simulink model "im_model_1"  (R2022b)
settings: Solver=VariableStepAuto  StartTime=0.0  StopTime=0.5  RelTol=1e-3
values from neighbouring files (symbols this model uses):
  B = 0.00825    [IM_System_1.m]    (also in IM_System_2.m; IM_System_3.m; IM_System_noPU_4p2p2kw.m; IM_System_noPU_4p2p2kw_1.m)
  D = Ls*Lr - Lm^2    (= 0.000595276666667)    [IM_System_1.m]    (also in IM_System_2.m; IM_System_3.m; IM_System_noPU_4p2p2kw.m; IM_System_noPU_4p2p2kw_1.m)
  J = 0.013    [IM_System_1.m]    (also in IM_System_2.m; IM_System_3.m; IM_System_noPU_4p2p2kw.m; IM_System_noPU_4p2p2kw_1.m)
  Lm = 0.245/3    (= 0.0816666666667)    [IM_System_1.m]    (also in IM_System_2.m; IM_System_3.m; IM_System_noPU_4p2p2kw.m; IM_System_noPU_4p2p2kw_1.m)
  Lr = Ls    (= 0.0852333333333)    [IM_System_1.m]    (also in IM_System_2.m; IM_System_3.m; IM_System_noPU_4p2p2kw.m; IM_System_noPU_4p2p2kw_1.m)
  Ls = 0.2557/3    (= 0.0852333333333)    [IM_System_1.m]    (also in IM_System_2.m; IM_System_3.m; IM_System_noPU_4p2p2kw.m; IM_System_noPU_4p2p2kw_1.m)
  pole = 4    [im_params.m]
  Rr = 1.83/3    (= 0.61)    [IM_System_1.m]    (also in IM_System_2.m; IM_System_3.m; IM_System_noPU_4p2p2kw.m; IM_System_noPU_4p2p2kw_1.m)
  Rs = 2.5/3    (= 0.833333333333)    [IM_System_1.m]    (also in IM_System_2.m; IM_System_3.m; IM_System_noPU_4p2p2kw.m; IM_System_noPU_4p2p2kw_1.m)
  w = w + iq_err*dt    (= -0.00016)    [IM_System_1.m]    (also in IM_System_2.m = -2e-05; IM_System_3.m = -2.2624e-05; IM_System_noPU_4p2p2kw.m = 0; IM_System_noPU_4p2p2kw_1.m = 0)
settings Model: Creator=jack  LastModifiedBy=jack

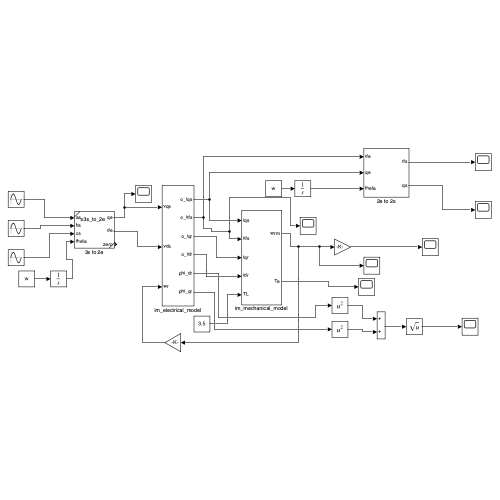
[thumbnail: Simulink's stored preview of the top-level diagram]
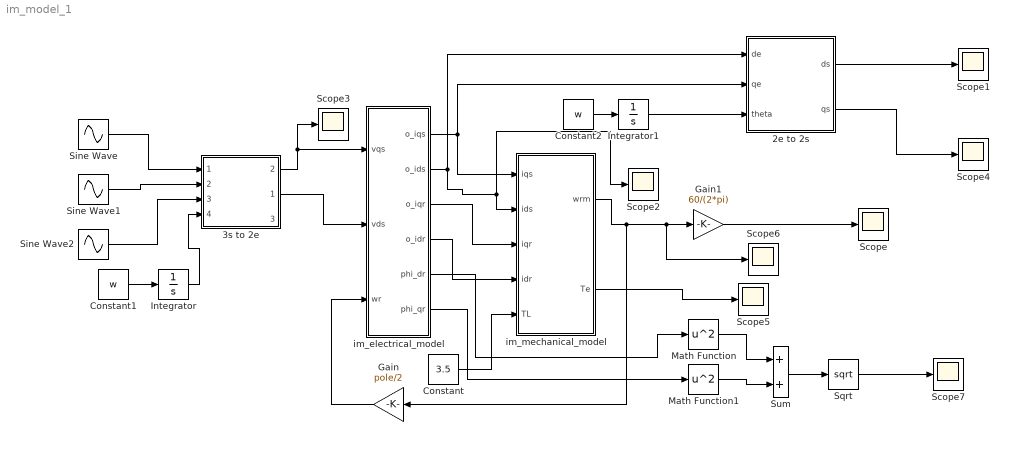
== system im_model_1 ==
  2e to 2s : Subsystem
  3s to 2e : Subsystem  ReferencedSubsystem=s3s_to_2e
      settings: PortSchema="{\"entries\":[{\"content\":{\"sides\":[{\"content\":{\"connectorIds\":[\"In1\",\"In2\",\"In3\",\"In4\"]},\"type\":\"ConnectorPlacement.EquallySpacedRectSide\",\"uuid\":\"f133be33-91f9-49ed-9811-9ea3b8c2cc59\"},{\"content\":{\"connectorIds\":[\"Out2\",\"Out1\",\"Out3\"],\"side\":\"RIGHT\"},\"type\":\"ConnectorPlacement.EquallySpacedRectSide\",\"uuid\":\"fabe9076-6ecf-4b28-bd28-ced1febe4377\"},{\"content\":{\"connectorIds\":[],\"side\":\"TOP\"},\"type\":\"ConnectorPlacement.EquallySpacedRectSide\",\"uuid\":\"329e6c38-eee0-47c4-808c-a4969678c6ab\"}]},\"type\":\"ConnectorPlacement.EquallySpacedConnector\",\"uuid\":\"55c86aad-84a3-4804-b18d-62086c80b5dc\"}],\"packageUris\":[\"http://schema.mathworks.com/mf0/Connector/R2020b\"],\"version\":\"1.0\"}"
  Constant : Constant  Value=3.5
  Constant1 : Constant  Value=w
  Constant2 : Constant  Value=w
  Gain : Gain  Gain=pole/2
  Gain1 : Gain  Gain=60/(2*pi)
  Integrator : Integrator
  Integrator1 : Integrator
  Math Function : Math  Operator=square
  Math Function1 : Math  Operator=square
  Scope{,1..7} (8 alike) : Scope
  Sine Wave : Sin  Amplitude=120*1.414  Frequency=w
  Sine Wave1 : Sin  Amplitude=120*1.414  Frequency=w  Phase=-2*pi/3
  Sine Wave2 : Sin  Amplitude=120*1.414  Frequency=w  Phase=2*pi/3
  Sqrt : Sqrt
  Sum : Sum
  im_electrical_model : Subsystem
  im_mechanical_model : Subsystem
  wires:
  Sine Wave/1 -> 3s to 2e/1
  Sine Wave1/1 -> 3s to 2e/2
  Sine Wave2/1 -> 3s to 2e/3
  3s to 2e/1 -> im_electrical_model/2(vds)
  im_electrical_model/1(o_iqs) -> 2e to 2s/2(qe), im_mechanical_model/1(iqs)
  im_electrical_model/2(o_ids) -> Scope2/1, im_mechanical_model/2(ids), 2e to 2s/1(de)
  im_electrical_model/3(o_iqr) -> im_mechanical_model/3(iqr)
  im_electrical_model/4(o_idr) -> im_mechanical_model/4(idr)
  Constant/1 -> im_mechanical_model/5(TL)
  im_mechanical_model/1(wrm) -> Gain/1, Scope6/1, Gain1/1
  Gain/1 -> im_electrical_model/3(wr)
  Constant1/1 -> Integrator/1
  Integrator/1 -> 3s to 2e/4
  3s to 2e/2 -> Scope3/1, im_electrical_model/1(vqs)
  Constant2/1 -> Integrator1/1
  Integrator1/1 -> 2e to 2s/3(theta)
  2e to 2s/1(ds) -> Scope1/1
  2e to 2s/2(qs) -> Scope4/1
  im_mechanical_model/2(Te) -> Scope5/1
  Gain1/1 -> Scope/1
  im_electrical_model/5(phi_dr) -> Math Function/1
  im_electrical_model/6(phi_qr) -> Math Function1/1
  Math Function/1 -> Sum/1
  Math Function1/1 -> Sum/2
  Sum/1 -> Sqrt/1
  Sqrt/1 -> Scope7/1

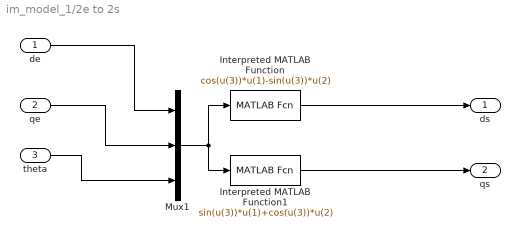
== system im_model_1/2e to 2s ==
  de : Inport
  qe : Inport  Port=2
  theta : Inport  Port=3
  Interpreted MATLAB Function : MATLABFcn  MATLABFcn=cos(u(3))*u(1)-sin(u(3))*u(2)
  Interpreted MATLAB Function1 : MATLABFcn  MATLABFcn=sin(u(3))*u(1)+cos(u(3))*u(2)
  Mux1 : Mux  Inputs=3
  ds : Outport
  qs : Outport  Port=2
  wires:
  theta/1 -> Mux1/3
  Interpreted MATLAB Function/1 -> ds/1
  qe/1 -> Mux1/2
  de/1 -> Mux1/1
  Interpreted MATLAB Function1/1 -> qs/1
  Mux1/1 -> Interpreted MATLAB Function/1, Interpreted MATLAB Function1/1

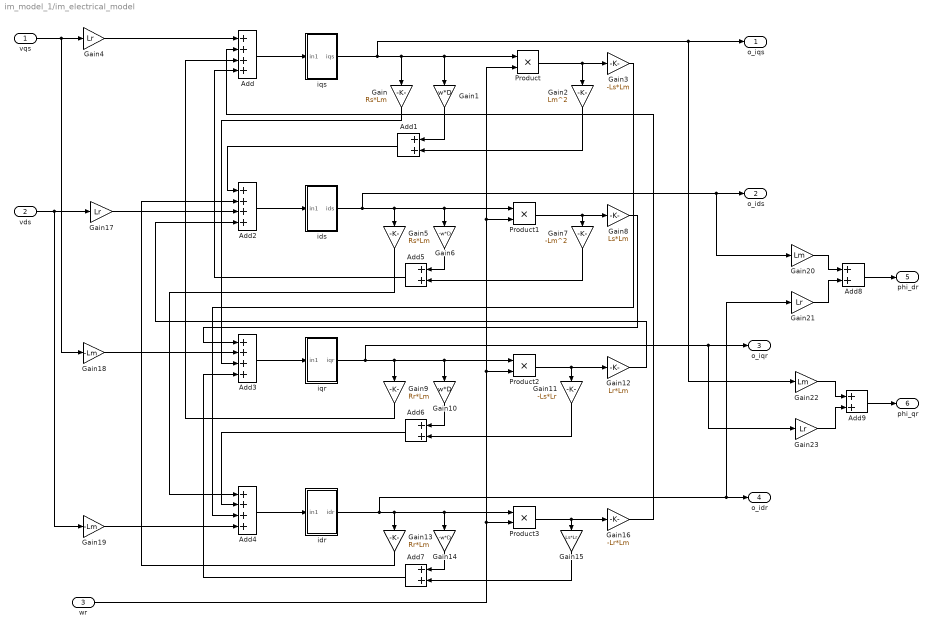
== system im_model_1/im_electrical_model ==
  vqs : Inport
  vds : Inport  Port=2
  wr : Inport  Port=3
  Add{,2..4} (4 alike) : Sum  Inputs=++++
  Add{1,5..9} (6 alike) : Sum
  Gain : Gain  Gain=Rs*Lm
  Gain1 : Gain  Gain=w*D
  Gain10 : Gain  Gain=w*D
  Gain11 : Gain  Gain=-Ls*Lr
  Gain12 : Gain  Gain=Lr*Lm
  Gain13 : Gain  Gain=Rr*Lm
  Gain14 : Gain  Gain=-w*D
  Gain15 : Gain  Gain=Ls*Lr
  Gain16 : Gain  Gain=-Lr*Lm
  Gain{4,17,21,23} (4 alike) : Gain  Gain=Lr
  Gain18 : Gain  Gain=-Lm
  Gain19 : Gain  Gain=-Lm
  Gain2 : Gain  Gain=Lm^2
  Gain20 : Gain  Gain=Lm
  Gain22 : Gain  Gain=Lm
  Gain3 : Gain  Gain=-Ls*Lm
  Gain5 : Gain  Gain=Rs*Lm
  Gain6 : Gain  Gain=-w*D
  Gain7 : Gain  Gain=-Lm^2
  Gain8 : Gain  Gain=Ls*Lm
  Gain9 : Gain  Gain=Rr*Lm
  Product{,1..3} (4 alike) : Product
  idr : Subsystem
  ids : Subsystem
  iqr : Subsystem
  iqs : Subsystem
  o_iqs : Outport
  o_ids : Outport  Port=2
  o_iqr : Outport  Port=3
  o_idr : Outport  Port=4
  phi_dr : Outport  Port=5
  phi_qr : Outport  Port=6
  wires:
  Add/1 -> iqs/1(in1)
  iqs/1(iqs) -> Gain22/1, o_iqs/1, Gain1/1, Product/1, Gain/1
  Gain1/1 -> Add1/1
  Product/1 -> Gain3/1, Gain2/1
  Gain2/1 -> Add1/2
  Gain/1 -> Add3/3
  Add1/1 -> Add2/1
  Gain4/1 -> Add/1
  vqs/1 -> Gain18/1, Gain4/1
  wr/1 -> Product3/2, Product2/2, Product1/2, Product/2
  Add2/1 -> ids/1(in1)
  Product1/1 -> Gain7/1, Gain8/1
  ids/1(ids) -> Gain20/1, o_ids/1, Gain5/1, Gain6/1, Product1/1
  Gain5/1 -> Add4/1
  Gain6/1 -> Add5/1
  Gain7/1 -> Add5/2
  Add5/1 -> Add/4
  Gain8/1 -> Add3/1
  iqr/1(iqr) -> Gain23/1, o_iqr/1, Gain9/1, Gain10/1, Product2/1
  Product2/1 -> Gain11/1, Gain12/1
  Gain10/1 -> Add6/1
  Gain11/1 -> Add6/2
  Add6/1 -> Add4/2
  Gain9/1 -> Add/3
  Gain12/1 -> Add2/4
  Add3/1 -> iqr/1(in1)
  idr/1(idr) -> Gain21/1, o_idr/1, Product3/1, Gain14/1, Gain13/1
  Gain14/1 -> Add7/1
  Gain15/1 -> Add7/2
  Product3/1 -> Gain15/1, Gain16/1
  Gain16/1 -> Add/2
  Add7/1 -> Add3/4
  Add4/1 -> idr/1(in1)
  Gain13/1 -> Add2/2
  Gain3/1 -> Add4/3
  vds/1 -> Gain19/1, Gain17/1
  Gain19/1 -> Add4/4
  Gain18/1 -> Add3/2
  Gain17/1 -> Add2/3
  Gain20/1 -> Add8/1
  Gain21/1 -> Add8/2
  Add8/1 -> phi_dr/1
  Gain23/1 -> Add9/2
  Gain22/1 -> Add9/1
  Add9/1 -> phi_qr/1

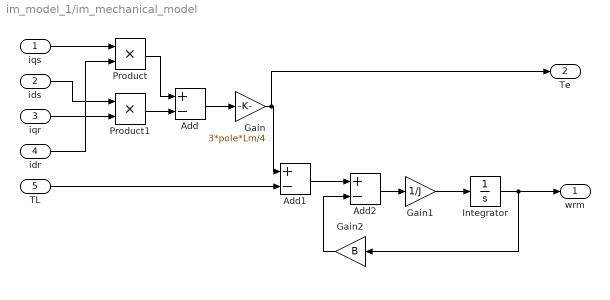
== system im_model_1/im_mechanical_model ==
  iqs : Inport
  ids : Inport  Port=2
  iqr : Inport  Port=3
  idr : Inport  Port=4
  TL : Inport  Port=5
  Add : Sum  Inputs=+-
  Add1 : Sum  Inputs=+-
  Add2 : Sum  Inputs=+-
  Gain : Gain  Gain=3*pole*Lm/4
  Gain1 : Gain  Gain=1/J
  Gain2 : Gain  Gain=B
  Integrator : Integrator
  Product : Product
  Product1 : Product
  wrm : Outport
  Te : Outport  Port=2
  wires:
  Add1/1 -> Add2/1
  iqr/1 -> Product1/2
  idr/1 -> Product/2
  TL/1 -> Add1/2
  iqs/1 -> Product/1
  Product/1 -> Add/1
  Add/1 -> Gain/1
  ids/1 -> Product1/1
  Add2/1 -> Gain1/1
  Gain1/1 -> Integrator/1
  Product1/1 -> Add/2
  Gain2/1 -> Add2/2
  Gain/1 -> Te/1, Add1/1
  Integrator/1 -> wrm/1, Gain2/1

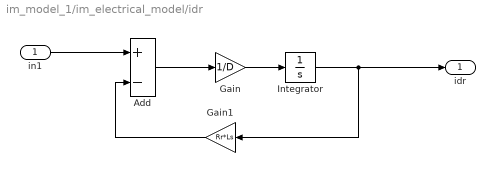
== system im_model_1/im_electrical_model/idr ==
  in1 : Inport
  Add : Sum  Inputs=+-
  Gain : Gain  Gain=1/D
  Gain1 : Gain  Gain=Rr*Ls
  Integrator : Integrator
  idr : Outport
  wires:
  in1/1 -> Add/1
  Gain1/1 -> Add/2
  Gain/1 -> Integrator/1
  Integrator/1 -> idr/1, Gain1/1
  Add/1 -> Gain/1

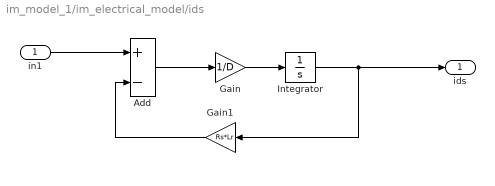
== system im_model_1/im_electrical_model/ids ==
  in1 : Inport
  Add : Sum  Inputs=+-
  Gain : Gain  Gain=1/D
  Gain1 : Gain  Gain=Rs*Lr
  Integrator : Integrator
  ids : Outport
  wires:
  Gain1/1 -> Add/2
  Gain/1 -> Integrator/1
  Add/1 -> Gain/1
  in1/1 -> Add/1
  Integrator/1 -> ids/1, Gain1/1

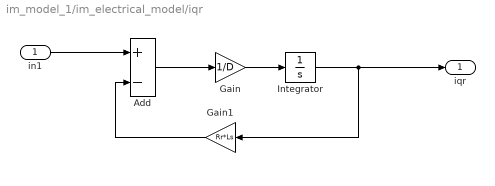
== system im_model_1/im_electrical_model/iqr ==
  in1 : Inport
  Add : Sum  Inputs=+-
  Gain : Gain  Gain=1/D
  Gain1 : Gain  Gain=Rr*Ls
  Integrator : Integrator
  iqr : Outport
  wires:
  in1/1 -> Add/1
  Gain/1 -> Integrator/1
  Gain1/1 -> Add/2
  Add/1 -> Gain/1
  Integrator/1 -> iqr/1, Gain1/1

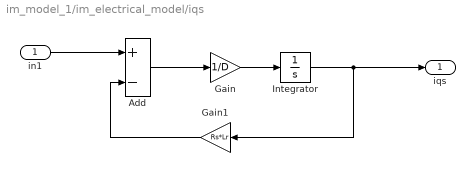
== system im_model_1/im_electrical_model/iqs ==
  in1 : Inport
  Add : Sum  Inputs=+-
  Gain : Gain  Gain=1/D
  Gain1 : Gain  Gain=Rs*Lr
  Integrator : Integrator
  iqs : Outport
  wires:
  Gain/1 -> Integrator/1
  Add/1 -> Gain/1
  in1/1 -> Add/1
  Gain1/1 -> Add/2
  Integrator/1 -> iqs/1, Gain1/1
